simulink model "lab2_2"  (R2020b)
settings: Solver=VariableStepAuto  StartTime=0.0  StopTime=10.0  RelTol=1e-10  AbsTol=1e-10
values from neighbouring files (symbols this model uses):
  La = 0.02    [lab1.m]
  Ra = 3    [lab1.m]
undefined symbols (not defined in the file or in its folder): g, km, M, ubar, ybar
libraries: cstblocks x1
settings Model: Creator=paulosga  LastModifiedBy=Adam Cassie

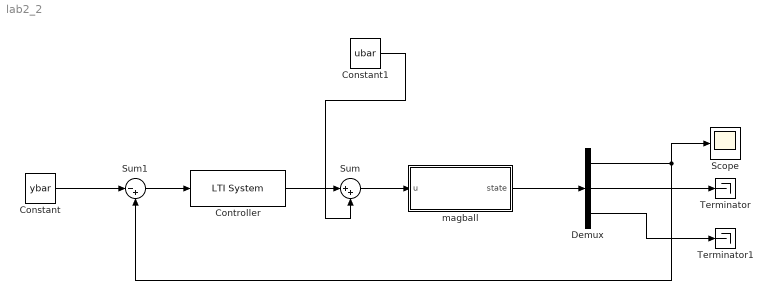
== system lab2_2 ==
  Constant : Constant  Value=ybar
  Constant1 : Constant  Value=ubar
  Controller : cstblocks/LTI System  sys=CONTROLLER  IC=[]
  Demux : Demux  Outputs=3
  Scope : Scope
  Sum : Sum  Inputs=|++
  Sum1 : Sum  Inputs=|-+
  Terminator : Terminator
  Terminator1 : Terminator
  magball : Subsystem
  wires:
  Controller/1 -> Sum/1
  Demux/1 -> Sum1/2, Scope/1
  Demux/3 -> Terminator1/1
  Demux/2 -> Terminator/1
  magball/1(state) -> Demux/1
  Constant1/1 -> Sum/2
  Sum1/1 -> Controller/1
  Constant/1 -> Sum1/1
  Sum/1 -> magball/1(u)

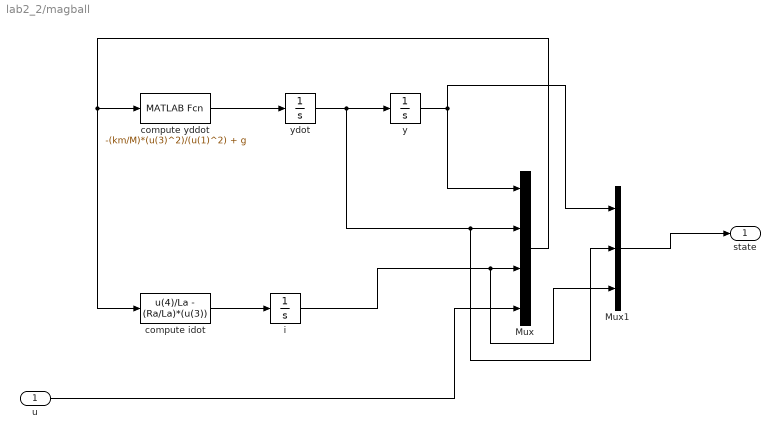
== system lab2_2/magball ==
  u : Inport
  Mux : Mux
  Mux1 : Mux  Inputs=3
  compute idot : MATLABFcn  MATLABFcn=u(4)/La - (Ra/La)*(u(3))
  compute yddot : MATLABFcn  MATLABFcn=-(km/M)*(u(3)^2)/(u(1)^2) + g
  i : Integrator
  y : Integrator  InitialCondition=0.15
  ydot : Integrator
  state : Outport
  wires:
  ydot/1 -> Mux1/2, Mux/2, y/1
  compute yddot/1 -> ydot/1
  compute idot/1 -> i/1
  Mux1/1 -> state/1
  y/1 -> Mux1/1, Mux/1
  Mux/1 -> compute idot/1, compute yddot/1
  i/1 -> Mux1/3, Mux/3
  u/1 -> Mux/4
